simulink model "manual_model_features"  (R2020b)
settings: Solver=VariableStepAuto  StartTime=0.0  StopTime=10.0  RelTol=1e-3
undefined symbols (not defined in the file): sigbuilder_block
libraries: simulink x141
(part 2 of 3)

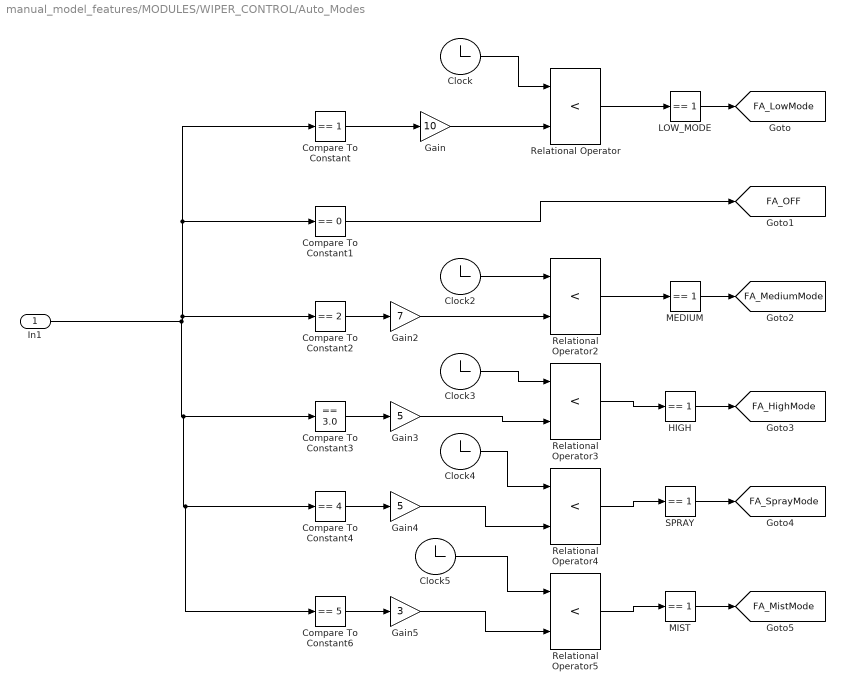
== system manual_model_features/MODULES/WIPER_CONTROL/Auto_Modes ==
  In1 : Inport
  Clock{,2..5} (5 alike) : Clock
      settings: Decimation=5
  Compare To Constant : simulink/Logic and Bit Operations/Compare To Constant  relop===  const=1  OutDataTypeStr=boolean
  Compare To Constant1 : simulink/Logic and Bit Operations/Compare To Constant  relop===  const=0  OutDataTypeStr=boolean
  Compare To Constant2 : simulink/Logic and Bit Operations/Compare To Constant  relop===  const=2  OutDataTypeStr=boolean
  Compare To Constant3 : simulink/Logic and Bit Operations/Compare To Constant  relop===  const=3.0  OutDataTypeStr=boolean
  Compare To Constant4 : simulink/Logic and Bit Operations/Compare To Constant  relop===  const=4  OutDataTypeStr=boolean
  Compare To Constant6 : simulink/Logic and Bit Operations/Compare To Constant  relop===  const=5  OutDataTypeStr=boolean
  Gain : Gain  Gain=10
  Gain2 : Gain  Gain=7
  Gain3 : Gain  Gain=5
  Gain4 : Gain  Gain=5
  Gain5 : Gain  Gain=3
  HIGH : simulink/Logic and Bit Operations/Compare To Constant  relop===  const=1  OutDataTypeStr=boolean
  LOW_MODE : simulink/Logic and Bit Operations/Compare To Constant  relop===  const=1  OutDataTypeStr=boolean
  MEDIUM : simulink/Logic and Bit Operations/Compare To Constant  relop===  const=1  OutDataTypeStr=boolean
  MIST : simulink/Logic and Bit Operations/Compare To Constant  relop===  const=1  OutDataTypeStr=boolean
  Relational Operator{,2..5} (5 alike) : RelationalOperator  Operator=<  OutDataTypeStr=boolean  RndMeth=Simplest
  SPRAY : simulink/Logic and Bit Operations/Compare To Constant  relop===  const=1  OutDataTypeStr=boolean
  tag scope: FA_HighMode=global, FA_LowMode=global, FA_MediumMode=global, FA_MistMode=global, FA_OFF=global, FA_SprayMode=global
  wires:
  In1/1 -> Compare To Constant6/1, Compare To Constant4/1, Compare To Constant3/1, Compare To Constant2/1, Compare To Constant/1, Compare To Constant1/1
  Clock/1 -> Relational Operator/1
  Relational Operator/1 -> LOW_MODE/1
  Gain/1 -> Relational Operator/2
  Compare To Constant/1 -> Gain/1
  Clock2/1 -> Relational Operator2/1
  Gain2/1 -> Relational Operator2/2
  Compare To Constant2/1 -> Gain2/1
  Clock3/1 -> Relational Operator3/1
  Gain3/1 -> Relational Operator3/2
  Compare To Constant3/1 -> Gain3/1
  Gain4/1 -> Relational Operator4/2
  Clock4/1 -> Relational Operator4/1
  Compare To Constant4/1 -> Gain4/1
  LOW_MODE/1 -> [FA_LowMode]
  MEDIUM/1 -> [FA_MediumMode]
  Relational Operator2/1 -> MEDIUM/1
  HIGH/1 -> [FA_HighMode]
  Relational Operator3/1 -> HIGH/1
  SPRAY/1 -> [FA_SprayMode]
  Relational Operator4/1 -> SPRAY/1
  Compare To Constant1/1 -> [FA_OFF]
  Relational Operator5/1 -> MIST/1
  Gain5/1 -> Relational Operator5/2
  Clock5/1 -> Relational Operator5/1
  MIST/1 -> [FA_MistMode]
  Compare To Constant6/1 -> Gain5/1

== system manual_model_features/MODULES/WIPER_CONTROL/Back_Windshield ==
  Lamp : LampBlock

== system manual_model_features/MODULES/WIPER_CONTROL/Front_Windshield ==
  Enable : EnablePort
  Auto_Modes : Subsystem
  Manual_mode : Subsystem
  Rotary Switch : RotarySwitchBlock  Commented=on
      settings: Values={{'Off', 'Low', 'Medium', 'High', 'Spray', 'Manual', 'MistMode'}, [0 1 2 3 4 5 6]}
  wires:
  [FW_Modes] -> Manual_mode/1(In1), Auto_Modes/1(In1)

== system manual_model_features/MODULES/WIPER_CONTROL/Manual_mode ==
  In1 : Inport
  Bw30_60 : Logic  IconShape=distinctive  AllPortsSameDT=off  OutDataTypeStr=boolean
  Bw60_100 : Logic  IconShape=distinctive  AllPortsSameDT=off  OutDataTypeStr=boolean
  Compare To Constant1 : simulink/Logic and Bit Operations/Compare To Constant  relop=>  const=30  OutDataTypeStr=boolean
  Compare To Constant2 : simulink/Logic and Bit Operations/Compare To Constant  relop=<=  const=60  OutDataTypeStr=boolean
  Compare To Constant3 : simulink/Logic and Bit Operations/Compare To Constant  relop=>  const=60  OutDataTypeStr=boolean
  Compare To Constant4 : simulink/Logic and Bit Operations/Compare To Constant  relop=<=  const=100  OutDataTypeStr=boolean
  Display : Display
  LessThan30 : simulink/Logic and Bit Operations/Compare To Constant  relop=<=  const=30  OutDataTypeStr=boolean
  Slider : SliderBlock
  String Constant : StringConstant  String="\"Undefined!\""
  Switch : Switch  Criteria=u2 > Threshold  Threshold=5
  tag scope: FM_Bw30_60=global, FM_Bw60_100=global, FM_lessthan30=global
  wires:
  Compare To Constant1/1 -> Bw30_60/1
  Bw30_60/1 -> [FM_Bw30_60]
  [FC_ManualInput] -> Compare To Constant4/1, Compare To Constant3/1, Compare To Constant2/1, Compare To Constant1/1, LessThan30/1, Switch/1
  Compare To Constant4/1 -> Bw60_100/2
  LessThan30/1 -> [FM_lessthan30]
  Switch/1 -> Display/1
  Compare To Constant3/1 -> Bw60_100/1
  Bw60_100/1 -> [FM_Bw60_100]
  Compare To Constant2/1 -> Bw30_60/2
  In1/1 -> Switch/2
  String Constant/1 -> Switch/3

== system manual_model_features/MODULES/WIPER_CONTROL/Wiper_Control ==
  Inport : Inport
  AND : Logic  IconShape=distinctive  AllPortsSameDT=off  OutDataTypeStr=boolean
  AND1 : Logic  IconShape=distinctive  AllPortsSameDT=off  OutDataTypeStr=boolean
  Atomic Subsystem : Subsystem  TreatAsAtomicUnit=on
  Atomic Subsystem1 : Subsystem  TreatAsAtomicUnit=on
  Back switch : SliderSwitchBlock  Commented=on
      settings: Values={{'Off', 'On'}, [0 1]}
  Back_Windshield : Subsystem  Commented=on  TreatAsAtomicUnit=on
  Front switch : SliderSwitchBlock  Commented=on
      settings: Values={{'Off', 'On'}, [0 1]}
  Front_Windshield : Subsystem  Commented=on  TreatAsAtomicUnit=on
  wires:
  Inport/1 -> AND1/2, AND/2
  [WC_FrontS] -> AND/1
  [WC_BackS] -> AND1/1
  AND1/1 -> Atomic Subsystem/1(Inport)
  AND/1 -> Atomic Subsystem1/1(Inport)

== system manual_model_features/MODULES/system/Automatic_Door_lock ==
  note: roof light
  AND : Logic  IconShape=distinctive  AllPortsSameDT=off  OutDataTypeStr=boolean
  Constant : Constant
  Display : Display
  Display1 : Display
  Display2 : Display
  If : If  IfExpression=u1>=13  ElseIfExpressions=u1<13  ShowElse=off
  If Action Subsystem : Subsystem  TreatAsAtomicUnit=on
  If Action Subsystem1 : Subsystem  TreatAsAtomicUnit=on
  OR : Logic  Operator=OR  IconShape=distinctive  AllPortsSameDT=off  OutDataTypeStr=boolean
  reset : Constant  Value=0
  Out1 : Outport
  wires:
  If Action Subsystem1/1(Out1) -> OR/2
  If Action Subsystem/1(Out1) -> OR/1
  [accln] -> Display/1, If/1
  Constant/1 -> If Action Subsystem/1(In1)
  [ADl_Ignition_System] -> Display1/1, AND/1
  reset/1 -> If Action Subsystem1/1(In1)
  If/2 -> If Action Subsystem1/Action
  If/1 -> If Action Subsystem/Action
  OR/1 -> AND/2
  AND/1 -> Display2/1, Out1/1

== system manual_model_features/MODULES/system/delay system door lock and interior light subsystem ==
  AND : Logic  Inputs=5  IconShape=distinctive  AllPortsSameDT=off  OutDataTypeStr=boolean
  AND1 : Logic  Inputs=4  IconShape=distinctive  AllPortsSameDT=off  OutDataTypeStr=boolean
  Add : Sum
  Compare To Constant : simulink/Logic and Bit Operations/Compare To Constant  relop===  const=0  OutDataTypeStr=boolean
  Constant4 : Constant  Value=0
  Constant5 : Constant  Value=0
  Data Type Conversion : DataTypeConversion
  Delay1 : Delay  DelayLength=1
  Display : Display
  Display1 : Display
  Repeating Sequence Stair : simulink/Sources/Repeating Sequence Stair  OutValues=[1 1]  tsamp=-1  OutMin=[]  OutMax=[]  OutDataTypeStr=double  OutputDataTypeScalingMode=double  OutDataType=fixdt(0,8)  ConRadixGroup=Best Precision: Vector-wise  OutScaling=2^-12
  Scope : Scope
  Switch : Switch  Threshold=5
  Switch1 : Switch
  Out1 : Outport
  tag scope: D_Sys_roof=global
  wires:
  Switch1/1 -> Scope/1, Out1/1, Delay1/1, Display/1
  [D_sys_antilock] -> AND/5
  Repeating Sequence Stair/1 -> Switch1/2
  Delay1/1 -> Add/2
  Constant5/1 -> Switch1/3
  Constant4/1 -> Switch/1
  Add/1 -> Switch/2, Switch/3
  Switch/1 -> Switch1/1
  AND/1 -> Data Type Conversion/1
  [D_sys_Door3] -> AND1/3, AND/3
  [D_sys_Door4] -> AND1/4, AND/4
  AND1/1 -> Compare To Constant/1
  [D_sys_Door1] -> AND1/1, AND/1
  [D_sys_Door2] -> AND1/2, AND/2
  Compare To Constant/1 -> [D_Sys_roof], Display1/1
  Data Type Conversion/1 -> Add/1

== system manual_model_features/MODULES/	POWER_WINDOW/Subsystem4/Front_left_subsystem ==
  lock/unlock : Inport
  In_fl_b : Inport  Port=2
  In_fl_Dc : Inport  Port=3
  object : Inport  Port=4
  Enable : EnablePort
  AND : Logic  IconShape=distinctive  AllPortsSameDT=off  OutDataTypeStr=boolean
  Compare To Constant1 : simulink/Logic and Bit Operations/Compare To Constant  relop===  const=1  OutDataTypeStr=boolean
  Display : Display
  Display1 : Display
  Scope : Scope  NumInputPorts=2
  Switch_lock_unlock : Switch  Criteria=u2 > Threshold
  check_ip : Constant
  decision_Box : Stateflow chart  TreatAsAtomicUnit=on
  inp_data : Logic  Operator=NXOR  IconShape=distinctive  AllPortsSameDT=off  OutDataTypeStr=boolean
  or1 : Logic  Operator=NXOR  IconShape=distinctive  AllPortsSameDT=off  OutDataTypeStr=boolean
  Outport : Outport
  Outport1 : Outport  Port=2
  tag scope: A=global
  wires:
  In_fl_b/1 -> AND/1
  check_ip/1 -> or1/1
  Switch_lock_unlock/1 -> [b1]
  Compare To Constant1/1 -> or1/2
  [b1] -> Display/1
  decision_Box/1(op1) -> Outport1/1, Switch_lock_unlock/3, Switch_lock_unlock/1, Scope/2, [A]
  decision_Box/2(warning) -> Outport/1, Scope/1
  object/1 -> decision_Box/2(data1)
  AND/1 -> inp_data/2  "res"
  or1/1 -> inp_data/1
  lock/unlock/1 -> AND/2, Switch_lock_unlock/2
  [A] -> Display1/1
  inp_data/1 -> decision_Box/1(data)
  In_fl_Dc/1 -> Compare To Constant1/1

== system manual_model_features/MODULES/	POWER_WINDOW/Subsystem4/Rear_right_Subsystem ==
  lock/unlock : Inport
  In2 : Inport  Port=2
  In3 : Inport  Port=3
  object : Inport  Port=4
  Enable : EnablePort
  Chart : Stateflow chart  TreatAsAtomicUnit=on
  Compare To Constant1 : simulink/Logic and Bit Operations/Compare To Constant  relop===  const=3  OutDataTypeStr=boolean
  Constant1 : Constant  Value=3
  Display2 : Display
  Display3 : Display
  Scope : Scope  NumInputPorts=2
  Switch : Switch  Criteria=u2 > Threshold
  or1 : Logic  Operator=NXOR  IconShape=distinctive  AllPortsSameDT=off  OutDataTypeStr=boolean
  or2 : Logic  IconShape=distinctive  AllPortsSameDT=off  OutDataTypeStr=boolean
  or3 : Logic  Operator=NXOR  IconShape=distinctive  AllPortsSameDT=off  OutDataTypeStr=boolean
  Outport : Outport
  Outport1 : Outport  Port=2
  tag scope: c=global
  wires:
  Constant1/1 -> or1/1
  [b3] -> Display2/1
  Compare To Constant1/1 -> or1/2
  Switch/1 -> [b3]
  lock/unlock/1 -> or2/2, Switch/2
  Chart/2(warning) -> Scope/1, Outport/1  "ss3"
  object/1 -> Chart/2(data1)
  or1/1 -> or3/2
  or2/1 -> or3/1  "res"
  or3/1 -> Chart/1(data)
  [c] -> Display3/1
  Chart/1(op1) -> Outport1/1, [c], Scope/2, Switch/3, Switch/1
  In2/1 -> or2/1
  In3/1 -> Compare To Constant1/1

== system manual_model_features/MODULES/	POWER_WINDOW/Subsystem4/driver_control_Subsystem ==
  In1 : Inport
  object : Inport  Port=2
  Enable : EnablePort
  Chart : Stateflow chart  TreatAsAtomicUnit=on
  Display4 : Display
  Scope : Scope  NumInputPorts=2
  Outport : Outport
  Outport1 : Outport  Port=2
  tag scope: d=global
  wires:
  Chart/2(warning) -> Outport/1, Scope/1  "ss4"
  object/1 -> Chart/2(data1)
  In1/1 -> Chart/1(data)
  [d] -> Display4/1
  Chart/1(op1) -> Outport1/1, [d], Scope/2

== system manual_model_features/MODULES/	POWER_WINDOW/Subsystem4/rear_left_Subsystem ==
  lock/unlock : Inport
  In2 : Inport  Port=2
  In3 : Inport  Port=3
  object : Inport  Port=4
  Enable : EnablePort
  Chart : Stateflow chart  TreatAsAtomicUnit=on
  Compare To Constant2 : simulink/Logic and Bit Operations/Compare To Constant  relop===  const=2  OutDataTypeStr=boolean
  Constant1 : Constant  Value=2
  Display1 : Display
  Display2 : Display
  Scope : Scope  NumInputPorts=2
  Switch1 : Switch  Criteria=u2 > Threshold
  or1 : Logic  Operator=NXOR  IconShape=distinctive  AllPortsSameDT=off  OutDataTypeStr=boolean
  or2 : Logic  Operator=NXOR  IconShape=distinctive  AllPortsSameDT=off  OutDataTypeStr=boolean
  or3 : Logic  IconShape=distinctive  AllPortsSameDT=off  OutDataTypeStr=boolean
  Outport : Outport
  Outport1 : Outport  Port=2
  tag scope: b=global
  wires:
  [b2] -> Display1/1
  Constant1/1 -> or2/1
  Compare To Constant2/1 -> or2/2
  Switch1/1 -> [b2]
  lock/unlock/1 -> Switch1/2, or3/2
  object/1 -> Chart/2(data1)
  Chart/2(warning) -> Outport/1, Scope/1  "ss2"
  or3/1 -> or1/1  "res"
  or2/1 -> or1/2
  or1/1 -> Chart/1(data)
  [b] -> Display2/1
  Chart/1(op1) -> Outport1/1, [b], Switch1/3, Switch1/1, Scope/2
  In2/1 -> or3/1
  In3/1 -> Compare To Constant2/1

== system manual_model_features/MODULES/AirBagSystem/FrontAirBagActivation/DriverFrontAirBagActive ==
  In1 : Inport
  Trigger : TriggerPort  VariantControl=(inherit)
  Constant : Constant
  Constant1 : Constant
  Constant2 : Constant
  Relational Operator : RelationalOperator  Operator===  OutDataTypeStr=boolean  RndMeth=Simplest
  Relational Operator1 : RelationalOperator  Operator===  OutDataTypeStr=boolean  RndMeth=Simplest
  Relational Operator2 : RelationalOperator  Operator===  OutDataTypeStr=boolean  RndMeth=Simplest
  tag scope: DriverAB=global, DriverDoor=global, FuelLock=global
  wires:
  In1/1 -> Relational Operator2/1, Relational Operator1/1, Relational Operator/1
  Constant/1 -> Relational Operator/2
  Constant1/1 -> Relational Operator1/2
  Constant2/1 -> Relational Operator2/2
  Relational Operator/1 -> [DriverAB]
  Relational Operator1/1 -> [DriverDoor]
  Relational Operator2/1 -> [FuelLock]

== system manual_model_features/MODULES/AirBagSystem/FrontAirBagActivation/LeftFrontAirBagActive ==
  In2 : Inport
  Trigger : TriggerPort  VariantControl=(inherit)
  Constant : Constant
  Constant1 : Constant
  Constant2 : Constant
  Relational Operator : RelationalOperator  Operator===  OutDataTypeStr=boolean  RndMeth=Simplest
  Relational Operator1 : RelationalOperator  Operator===  OutDataTypeStr=boolean  RndMeth=Simplest
  Relational Operator2 : RelationalOperator  Operator===  OutDataTypeStr=boolean  RndMeth=Simplest
  tag scope: FuelLock1=global, LeftFront=global, LeftFrontDoor=global
  wires:
  Constant1/1 -> Relational Operator1/2
  In2/1 -> Relational Operator2/1, Relational Operator1/1, Relational Operator/1
  Constant2/1 -> Relational Operator2/2
  Constant/1 -> Relational Operator/2
  Relational Operator/1 -> [LeftFront]
  Relational Operator1/1 -> [LeftFrontDoor]
  Relational Operator2/1 -> [FuelLock1]

== system manual_model_features/MODULES/AirBagSystem/FrontAirBagActivation/LeftRearAirBagActive ==
  In1 : Inport
  Trigger : TriggerPort  VariantControl=(inherit)
  Constant : Constant
  Constant1 : Constant
  Constant2 : Constant
  Relational Operator : RelationalOperator  Operator===  OutDataTypeStr=boolean  RndMeth=Simplest
  Relational Operator1 : RelationalOperator  Operator===  OutDataTypeStr=boolean  RndMeth=Simplest
  Relational Operator2 : RelationalOperator  Operator===  OutDataTypeStr=boolean  RndMeth=Simplest
  tag scope: FuelLock2=global, RearLeft=global, RearLeftDoor=global
  wires:
  Constant1/1 -> Relational Operator1/2
  In1/1 -> Relational Operator2/1, Relational Operator1/1, Relational Operator/1
  Constant2/1 -> Relational Operator2/2
  Constant/1 -> Relational Operator/2
  Relational Operator/1 -> [RearLeft]
  Relational Operator1/1 -> [RearLeftDoor]
  Relational Operator2/1 -> [FuelLock2]

== system manual_model_features/MODULES/AirBagSystem/FrontAirBagActivation/RightRearAirBagActive ==
  In2 : Inport
  Trigger : TriggerPort  VariantControl=(inherit)
  Constant : Constant
  Constant1 : Constant
  Constant2 : Constant
  Relational Operator : RelationalOperator  Operator===  OutDataTypeStr=boolean  RndMeth=Simplest
  Relational Operator1 : RelationalOperator  Operator===  OutDataTypeStr=boolean  RndMeth=Simplest
  Relational Operator2 : RelationalOperator  Operator===  OutDataTypeStr=boolean  RndMeth=Simplest
  tag scope: FuelLock3=global, RearRight=global, RearRightDoor=global
  wires:
  Constant1/1 -> Relational Operator1/2
  In2/1 -> Relational Operator2/1, Relational Operator1/1, Relational Operator/1
  Constant2/1 -> Relational Operator2/2
  Constant/1 -> Relational Operator/2
  Relational Operator/1 -> [RearRight]
  Relational Operator1/1 -> [RearRightDoor]
  Relational Operator2/1 -> [FuelLock3]

== system manual_model_features/MODULES/AirBagSystem/SideAirBagActivation/DriverSideAirBagActive ==
  In1 : Inport
  Trigger : TriggerPort  VariantControl=(inherit)
  Constant : Constant
  Constant1 : Constant
  Constant2 : Constant
  Relational Operator : RelationalOperator  Operator===  OutDataTypeStr=boolean  RndMeth=Simplest
  Relational Operator1 : RelationalOperator  Operator===  OutDataTypeStr=boolean  RndMeth=Simplest
  Relational Operator2 : RelationalOperator  Operator===  OutDataTypeStr=boolean  RndMeth=Simplest
  tag scope: DriverABSide=global, DriverDoorSide=global, FuelLockSide=global
  wires:
  In1/1 -> Relational Operator2/1, Relational Operator1/1, Relational Operator/1
  Constant/1 -> Relational Operator/2
  Constant1/1 -> Relational Operator1/2
  Constant2/1 -> Relational Operator2/2
  Relational Operator/1 -> [DriverABSide]
  Relational Operator1/1 -> [DriverDoorSide]
  Relational Operator2/1 -> [FuelLockSide]

== system manual_model_features/MODULES/AirBagSystem/SideAirBagActivation/LeftFronrSeatAirBagActive ==
  In2 : Inport
  Trigger : TriggerPort  VariantControl=(inherit)
  Constant : Constant
  Constant1 : Constant
  Constant2 : Constant
  Relational Operator : RelationalOperator  Operator===  OutDataTypeStr=boolean  RndMeth=Simplest
  Relational Operator1 : RelationalOperator  Operator===  OutDataTypeStr=boolean  RndMeth=Simplest
  Relational Operator2 : RelationalOperator  Operator===  OutDataTypeStr=boolean  RndMeth=Simplest
  tag scope: FuelLockSide1=global, LeftFrontDoorSide=global, LeftFrontSide=global
  wires:
  Constant1/1 -> Relational Operator1/2
  In2/1 -> Relational Operator2/1, Relational Operator1/1, Relational Operator/1
  Constant2/1 -> Relational Operator2/2
  Constant/1 -> Relational Operator/2
  Relational Operator/1 -> [LeftFrontSide]
  Relational Operator1/1 -> [LeftFrontDoorSide]
  Relational Operator2/1 -> [FuelLockSide1]

== system manual_model_features/MODULES/AirBagSystem/SideAirBagActivation/LeftRearAirBagActive ==
  In1 : Inport
  Trigger : TriggerPort  VariantControl=(inherit)
  Constant : Constant
  Constant1 : Constant
  Constant2 : Constant
  Relational Operator : RelationalOperator  Operator===  OutDataTypeStr=boolean  RndMeth=Simplest
  Relational Operator1 : RelationalOperator  Operator===  OutDataTypeStr=boolean  RndMeth=Simplest
  Relational Operator2 : RelationalOperator  Operator===  OutDataTypeStr=boolean  RndMeth=Simplest
  tag scope: FuelLockSide2=global, RearLeftDoorSide=global, RearLeftSide=global
  wires:
  Constant1/1 -> Relational Operator1/2
  In1/1 -> Relational Operator2/1, Relational Operator1/1, Relational Operator/1
  Constant2/1 -> Relational Operator2/2
  Constant/1 -> Relational Operator/2
  Relational Operator1/1 -> [RearLeftDoorSide]
  Relational Operator2/1 -> [FuelLockSide2]
  Relational Operator/1 -> [RearLeftSide]

== system manual_model_features/MODULES/AirBagSystem/SideAirBagActivation/RightRearAirBagActive ==
  In2 : Inport
  Trigger : TriggerPort  VariantControl=(inherit)
  Constant : Constant
  Constant1 : Constant
  Constant2 : Constant
  Relational Operator : RelationalOperator  Operator===  OutDataTypeStr=boolean  RndMeth=Simplest
  Relational Operator1 : RelationalOperator  Operator===  OutDataTypeStr=boolean  RndMeth=Simplest
  Relational Operator2 : RelationalOperator  Operator===  OutDataTypeStr=boolean  RndMeth=Simplest
  tag scope: FuelLockSide3=global, RearRightDoorSide=global, RearRightSide=global
  wires:
  Constant1/1 -> Relational Operator1/2
  In2/1 -> Relational Operator2/1, Relational Operator1/1, Relational Operator/1
  Constant2/1 -> Relational Operator2/2
  Constant/1 -> Relational Operator/2
  Relational Operator/1 -> [RearRightSide]
  Relational Operator1/1 -> [RearRightDoorSide]
  Relational Operator2/1 -> [FuelLockSide3]

== system manual_model_features/MODULES/AirBagSystem2/FrontAirBagActivation/DriverFrontAirBagActive ==
  In1 : Inport
  Trigger : TriggerPort  VariantControl=(inherit)
  Constant : Constant
  Constant1 : Constant
  Constant2 : Constant
  DriverDoorUnlock : LampBlock
  DriverFront : LampBlock
  FuelLock : LampBlock
  Relational Operator : RelationalOperator  Operator===  OutDataTypeStr=boolean  RndMeth=Simplest
  Relational Operator1 : RelationalOperator  Operator===  OutDataTypeStr=boolean  RndMeth=Simplest
  Relational Operator2 : RelationalOperator  Operator===  OutDataTypeStr=boolean  RndMeth=Simplest
  wires:
  In1/1 -> Relational Operator2/1, Relational Operator1/1, Relational Operator/1
  Constant/1 -> Relational Operator/2
  Constant1/1 -> Relational Operator1/2
  Constant2/1 -> Relational Operator2/2

== system manual_model_features/MODULES/AirBagSystem2/FrontAirBagActivation/LeftFrontAirBagActive ==
  In2 : Inport
  Trigger : TriggerPort  VariantControl=(inherit)
  Constant : Constant
  Constant1 : Constant
  Constant2 : Constant
  FuelLock : LampBlock
  LeftDoorUnlock : LampBlock
  LeftFront : LampBlock
  Relational Operator : RelationalOperator  Operator===  OutDataTypeStr=boolean  RndMeth=Simplest
  Relational Operator1 : RelationalOperator  Operator===  OutDataTypeStr=boolean  RndMeth=Simplest
  Relational Operator2 : RelationalOperator  Operator===  OutDataTypeStr=boolean  RndMeth=Simplest
  wires:
  Constant1/1 -> Relational Operator1/2
  In2/1 -> Relational Operator2/1, Relational Operator1/1, Relational Operator/1
  Constant2/1 -> Relational Operator2/2
  Constant/1 -> Relational Operator/2

== system manual_model_features/MODULES/AirBagSystem2/FrontAirBagActivation/LeftRearAirBagActive ==
  In1 : Inport
  Trigger : TriggerPort  VariantControl=(inherit)
  Constant : Constant
  Constant1 : Constant
  Constant2 : Constant
  FuelLock : LampBlock
  LeftRear : LampBlock
  LeftRearDoorUnlock : LampBlock
  Relational Operator : RelationalOperator  Operator===  OutDataTypeStr=boolean  RndMeth=Simplest
  Relational Operator1 : RelationalOperator  Operator===  OutDataTypeStr=boolean  RndMeth=Simplest
  Relational Operator2 : RelationalOperator  Operator===  OutDataTypeStr=boolean  RndMeth=Simplest
  wires:
  Constant1/1 -> Relational Operator1/2
  In1/1 -> Relational Operator2/1, Relational Operator1/1, Relational Operator/1
  Constant2/1 -> Relational Operator2/2
  Constant/1 -> Relational Operator/2

== system manual_model_features/MODULES/AirBagSystem2/FrontAirBagActivation/RightRearAirBagActive ==
  In2 : Inport
  Trigger : TriggerPort  VariantControl=(inherit)
  Constant : Constant
  Constant1 : Constant
  Constant2 : Constant
  FuelLock : LampBlock
  Relational Operator : RelationalOperator  Operator===  OutDataTypeStr=boolean  RndMeth=Simplest
  Relational Operator1 : RelationalOperator  Operator===  OutDataTypeStr=boolean  RndMeth=Simplest
  Relational Operator2 : RelationalOperator  Operator===  OutDataTypeStr=boolean  RndMeth=Simplest
  RightRear : LampBlock
  RightRearDoorUnlock : LampBlock
  wires:
  Constant1/1 -> Relational Operator1/2
  In2/1 -> Relational Operator2/1, Relational Operator1/1, Relational Operator/1
  Constant2/1 -> Relational Operator2/2
  Constant/1 -> Relational Operator/2

== system manual_model_features/MODULES/AirBagSystem2/FrontAirBagActivation1/DriverSideAirBagActive ==
  In1 : Inport
  Trigger : TriggerPort  VariantControl=(inherit)
  Constant : Constant
  Constant1 : Constant
  Constant2 : Constant
  DriverDoorUnlock : LampBlock
  DriverFront : LampBlock
  FuelLock : LampBlock
  Relational Operator : RelationalOperator  Operator===  OutDataTypeStr=boolean  RndMeth=Simplest
  Relational Operator1 : RelationalOperator  Operator===  OutDataTypeStr=boolean  RndMeth=Simplest
  Relational Operator2 : RelationalOperator  Operator===  OutDataTypeStr=boolean  RndMeth=Simplest
  Out1 : Outport
  wires:
  In1/1 -> Relational Operator2/1, Relational Operator1/1, Relational Operator/1
  Constant/1 -> Relational Operator/2
  Constant1/1 -> Relational Operator1/2
  Constant2/1 -> Relational Operator2/2

== system manual_model_features/MODULES/AirBagSystem2/FrontAirBagActivation1/LeftFronrSeatAirBagActive ==
  In2 : Inport
  Trigger : TriggerPort  VariantControl=(inherit)
  Constant : Constant
  Constant1 : Constant
  Constant2 : Constant
  FuelLock : LampBlock
  LeftDoorUnlock : LampBlock
  LeftFront : LampBlock
  Relational Operator : RelationalOperator  Operator===  OutDataTypeStr=boolean  RndMeth=Simplest
  Relational Operator1 : RelationalOperator  Operator===  OutDataTypeStr=boolean  RndMeth=Simplest
  Relational Operator2 : RelationalOperator  Operator===  OutDataTypeStr=boolean  RndMeth=Simplest
  wires:
  Constant1/1 -> Relational Operator1/2
  In2/1 -> Relational Operator2/1, Relational Operator1/1, Relational Operator/1
  Constant2/1 -> Relational Operator2/2
  Constant/1 -> Relational Operator/2

== system manual_model_features/MODULES/AirBagSystem2/FrontAirBagActivation1/LeftRearAirBagActive ==
  In1 : Inport
  Trigger : TriggerPort  VariantControl=(inherit)
  Constant : Constant
  Constant1 : Constant
  Constant2 : Constant
  FuelLock : LampBlock
  LeftRear : LampBlock
  LeftRearDoorUnlock : LampBlock
  Relational Operator : RelationalOperator  Operator===  OutDataTypeStr=boolean  RndMeth=Simplest
  Relational Operator1 : RelationalOperator  Operator===  OutDataTypeStr=boolean  RndMeth=Simplest
  Relational Operator2 : RelationalOperator  Operator===  OutDataTypeStr=boolean  RndMeth=Simplest
  wires:
  Constant1/1 -> Relational Operator1/2
  In1/1 -> Relational Operator2/1, Relational Operator1/1, Relational Operator/1
  Constant2/1 -> Relational Operator2/2
  Constant/1 -> Relational Operator/2

== system manual_model_features/MODULES/AirBagSystem2/FrontAirBagActivation1/RightRearAirBagActive ==
  In2 : Inport
  Trigger : TriggerPort  VariantControl=(inherit)
  Constant : Constant
  Constant1 : Constant
  Constant2 : Constant
  FuelLock : LampBlock
  Relational Operator : RelationalOperator  Operator===  OutDataTypeStr=boolean  RndMeth=Simplest
  Relational Operator1 : RelationalOperator  Operator===  OutDataTypeStr=boolean  RndMeth=Simplest
  Relational Operator2 : RelationalOperator  Operator===  OutDataTypeStr=boolean  RndMeth=Simplest
  RightRear : LampBlock
  RightRearDoorUnlock : LampBlock
  wires:
  Constant1/1 -> Relational Operator1/2
  In2/1 -> Relational Operator2/1, Relational Operator1/1, Relational Operator/1
  Constant2/1 -> Relational Operator2/2
  Constant/1 -> Relational Operator/2

== system manual_model_features/MODULES/Door_System/AutomaticDoorLock/If Action Subsystem ==
  In1 : Inport
  Action Port : ActionPort
  Out1 : Outport
  wires:
  In1/1 -> Out1/1

== system manual_model_features/MODULES/Door_System/AutomaticDoorLock/If Action Subsystem1 ==
  In1 : Inport
  Action Port : ActionPort
  Out1 : Outport
  wires:
  In1/1 -> Out1/1

== system manual_model_features/MODULES/SeatRestraintSystem1/PowerLumbar/PowerSeat ==
  RearAdjust : Inport
  SeatAdjust : Inport  Port=2
  CushionAdjust : Inport  Port=3
  Enable : EnablePort
  ModeSelection==RearAdjust : Constant  Value=2
  Subsystem : Subsystem
  Subsystem1 : Subsystem
  Subsystem2 : Subsystem
  wires:
  RearAdjust/1 -> Subsystem/1(Rear_Adjust)
  ModeSelection==RearAdjust/1 -> Subsystem2/1(Mode_Check), Subsystem1/1(Mode_Check), Subsystem/2(Mode_Check)
  SeatAdjust/1 -> Subsystem1/2(Seat_Adjust)
  CushionAdjust/1 -> Subsystem2/2(CushionAdjust)

== system manual_model_features/MODULES/Subsystem2/Subsystem/Enabled Subsystem ==
  In1 : Inport
  Enable : EnablePort
  Outport : Outport
  wires:
  In1/1 -> Outport/1

== system manual_model_features/MODULES/Subsystem2/Subsystem1/Enabled Subsystem1 ==
  In1 : Inport
  Enable : EnablePort
  Outport : Outport
  wires:
  In1/1 -> Outport/1

== system manual_model_features/MODULES/Tire Pressure Monitoring System/TP_Monitoring/indicateHigh1 ==
  Enable : EnablePort
  Constant : Constant  Value=0
  Out1 : Outport
  wires:
  Constant/1 -> Out1/1

== system manual_model_features/MODULES/Tire Pressure Monitoring System/TP_Monitoring/indicateHigh2 ==
  Enable : EnablePort
  Constant : Constant  Value=0
  Out1 : Outport
  wires:
  Constant/1 -> Out1/1

== system manual_model_features/MODULES/Tire Pressure Monitoring System/TP_Monitoring/indicateHigh3 ==
  Enable : EnablePort
  Constant : Constant  Value=0
  Out1 : Outport
  wires:
  Constant/1 -> Out1/1

== system manual_model_features/MODULES/Tire Pressure Monitoring System/TP_Monitoring/indicateHigh4 ==
  Enable : EnablePort
  Constant : Constant  Value=0
  Out1 : Outport
  wires:
  Constant/1 -> Out1/1

== system manual_model_features/MODULES/Tire Pressure Monitoring System/TP_Monitoring/indicateLow1 ==
  Enable : EnablePort
  Constant : Constant
  Out1 : Outport
  wires:
  Constant/1 -> Out1/1

== system manual_model_features/MODULES/Tire Pressure Monitoring System/TP_Monitoring/indicateLow2 ==
  Enable : EnablePort
  Constant : Constant
  Out1 : Outport
  wires:
  Constant/1 -> Out1/1

== system manual_model_features/MODULES/Tire Pressure Monitoring System/TP_Monitoring/indicateLow3 ==
  Enable : EnablePort
  Constant : Constant
  Out1 : Outport
  wires:
  Constant/1 -> Out1/1

== system manual_model_features/MODULES/Tire Pressure Monitoring System/TP_Monitoring/indicateLow4 ==
  Enable : EnablePort
  Constant : Constant
  Out1 : Outport
  wires:
  Constant/1 -> Out1/1

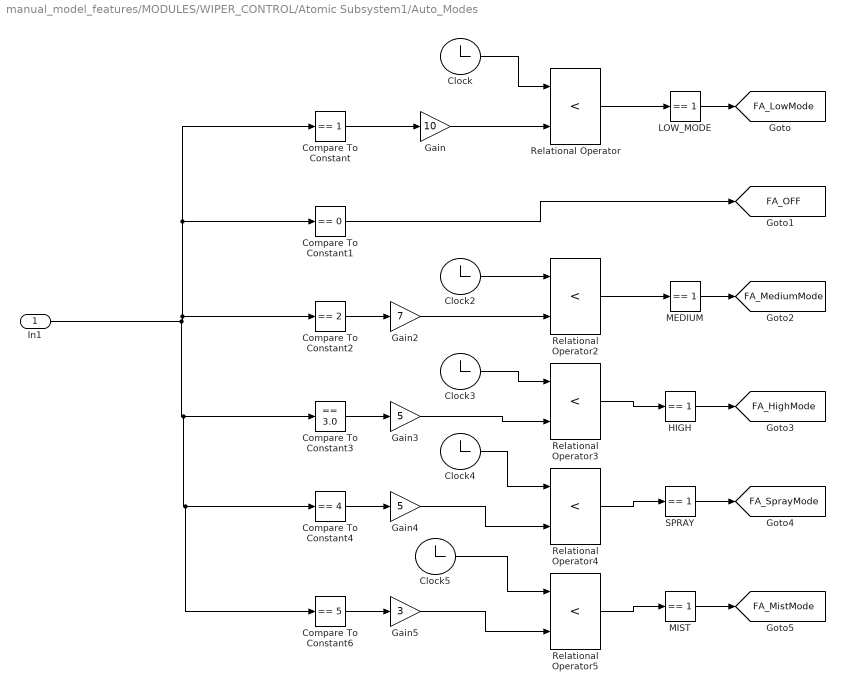
== system manual_model_features/MODULES/WIPER_CONTROL/Atomic Subsystem1/Auto_Modes ==
  In1 : Inport
  Clock{,2..5} (5 alike) : Clock
      settings: Decimation=5
  Compare To Constant : simulink/Logic and Bit Operations/Compare To Constant  relop===  const=1  OutDataTypeStr=boolean
  Compare To Constant1 : simulink/Logic and Bit Operations/Compare To Constant  relop===  const=0  OutDataTypeStr=boolean
  Compare To Constant2 : simulink/Logic and Bit Operations/Compare To Constant  relop===  const=2  OutDataTypeStr=boolean
  Compare To Constant3 : simulink/Logic and Bit Operations/Compare To Constant  relop===  const=3.0  OutDataTypeStr=boolean
  Compare To Constant4 : simulink/Logic and Bit Operations/Compare To Constant  relop===  const=4  OutDataTypeStr=boolean
  Compare To Constant6 : simulink/Logic and Bit Operations/Compare To Constant  relop===  const=5  OutDataTypeStr=boolean
  Gain : Gain  Gain=10
  Gain2 : Gain  Gain=7
  Gain3 : Gain  Gain=5
  Gain4 : Gain  Gain=5
  Gain5 : Gain  Gain=3
  HIGH : simulink/Logic and Bit Operations/Compare To Constant  relop===  const=1  OutDataTypeStr=boolean
  LOW_MODE : simulink/Logic and Bit Operations/Compare To Constant  relop===  const=1  OutDataTypeStr=boolean
  MEDIUM : simulink/Logic and Bit Operations/Compare To Constant  relop===  const=1  OutDataTypeStr=boolean
  MIST : simulink/Logic and Bit Operations/Compare To Constant  relop===  const=1  OutDataTypeStr=boolean
  Relational Operator{,2..5} (5 alike) : RelationalOperator  Operator=<  OutDataTypeStr=boolean  RndMeth=Simplest
  SPRAY : simulink/Logic and Bit Operations/Compare To Constant  relop===  const=1  OutDataTypeStr=boolean
  tag scope: FA_HighMode=global, FA_LowMode=global, FA_MediumMode=global, FA_MistMode=global, FA_OFF=global, FA_SprayMode=global
  wires:
  In1/1 -> Compare To Constant6/1, Compare To Constant4/1, Compare To Constant3/1, Compare To Constant2/1, Compare To Constant/1, Compare To Constant1/1
  Clock/1 -> Relational Operator/1
  Relational Operator/1 -> LOW_MODE/1
  Gain/1 -> Relational Operator/2
  Compare To Constant/1 -> Gain/1
  Clock2/1 -> Relational Operator2/1
  Gain2/1 -> Relational Operator2/2
  Compare To Constant2/1 -> Gain2/1
  Clock3/1 -> Relational Operator3/1
  Gain3/1 -> Relational Operator3/2
  Compare To Constant3/1 -> Gain3/1
  Gain4/1 -> Relational Operator4/2
  Clock4/1 -> Relational Operator4/1
  Compare To Constant4/1 -> Gain4/1
  LOW_MODE/1 -> [FA_LowMode]
  MEDIUM/1 -> [FA_MediumMode]
  Relational Operator2/1 -> MEDIUM/1
  HIGH/1 -> [FA_HighMode]
  Relational Operator3/1 -> HIGH/1
  SPRAY/1 -> [FA_SprayMode]
  Relational Operator4/1 -> SPRAY/1
  Compare To Constant1/1 -> [FA_OFF]
  Relational Operator5/1 -> MIST/1
  Gain5/1 -> Relational Operator5/2
  Clock5/1 -> Relational Operator5/1
  MIST/1 -> [FA_MistMode]
  Compare To Constant6/1 -> Gain5/1

== system manual_model_features/MODULES/WIPER_CONTROL/Atomic Subsystem1/Manual_mode ==
  In1 : Inport
  Bw30_60 : Logic  IconShape=distinctive  AllPortsSameDT=off  OutDataTypeStr=boolean
  Bw60_100 : Logic  IconShape=distinctive  AllPortsSameDT=off  OutDataTypeStr=boolean
  Compare To Constant1 : simulink/Logic and Bit Operations/Compare To Constant  relop=>  const=30  OutDataTypeStr=boolean
  Compare To Constant2 : simulink/Logic and Bit Operations/Compare To Constant  relop=<=  const=60  OutDataTypeStr=boolean
  Compare To Constant3 : simulink/Logic and Bit Operations/Compare To Constant  relop=>  const=60  OutDataTypeStr=boolean
  Compare To Constant4 : simulink/Logic and Bit Operations/Compare To Constant  relop=<=  const=100  OutDataTypeStr=boolean
  Display : Display
  LessThan30 : simulink/Logic and Bit Operations/Compare To Constant  relop=<=  const=30  OutDataTypeStr=boolean
  Slider : SliderBlock
  String Constant : StringConstant  String="\"Undefined!\""
  Switch : Switch  Criteria=u2 > Threshold  Threshold=5
  tag scope: FM_Bw30_60=global, FM_Bw60_100=global, FM_lessthan30=global
  wires:
  Compare To Constant1/1 -> Bw30_60/1
  Bw30_60/1 -> [FM_Bw30_60]
  [FC_ManualInput] -> Compare To Constant4/1, Compare To Constant3/1, Compare To Constant2/1, Compare To Constant1/1, LessThan30/1, Switch/1
  Compare To Constant4/1 -> Bw60_100/2
  LessThan30/1 -> [FM_lessthan30]
  Switch/1 -> Display/1
  Compare To Constant3/1 -> Bw60_100/1
  Bw60_100/1 -> [FM_Bw60_100]
  Compare To Constant2/1 -> Bw30_60/2
  In1/1 -> Switch/2
  String Constant/1 -> Switch/3

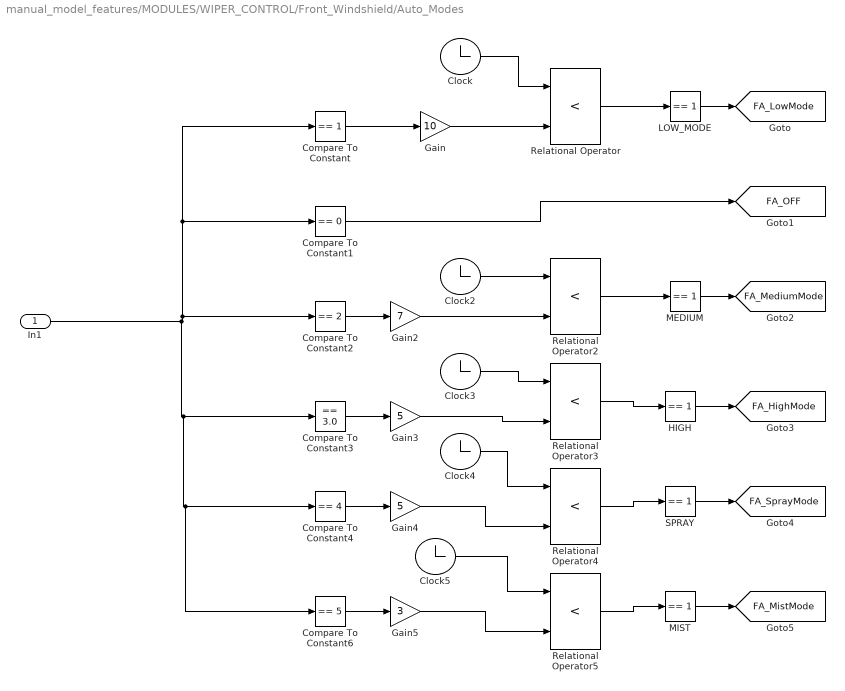
== system manual_model_features/MODULES/WIPER_CONTROL/Front_Windshield/Auto_Modes ==
  In1 : Inport
  Clock{,2..5} (5 alike) : Clock
      settings: Decimation=5
  Compare To Constant : simulink/Logic and Bit Operations/Compare To Constant  relop===  const=1  OutDataTypeStr=boolean
  Compare To Constant1 : simulink/Logic and Bit Operations/Compare To Constant  relop===  const=0  OutDataTypeStr=boolean
  Compare To Constant2 : simulink/Logic and Bit Operations/Compare To Constant  relop===  const=2  OutDataTypeStr=boolean
  Compare To Constant3 : simulink/Logic and Bit Operations/Compare To Constant  relop===  const=3.0  OutDataTypeStr=boolean
  Compare To Constant4 : simulink/Logic and Bit Operations/Compare To Constant  relop===  const=4  OutDataTypeStr=boolean
  Compare To Constant6 : simulink/Logic and Bit Operations/Compare To Constant  relop===  const=5  OutDataTypeStr=boolean
  Gain : Gain  Gain=10
  Gain2 : Gain  Gain=7
  Gain3 : Gain  Gain=5
  Gain4 : Gain  Gain=5
  Gain5 : Gain  Gain=3
  HIGH : simulink/Logic and Bit Operations/Compare To Constant  relop===  const=1  OutDataTypeStr=boolean
  LOW_MODE : simulink/Logic and Bit Operations/Compare To Constant  relop===  const=1  OutDataTypeStr=boolean
  MEDIUM : simulink/Logic and Bit Operations/Compare To Constant  relop===  const=1  OutDataTypeStr=boolean
  MIST : simulink/Logic and Bit Operations/Compare To Constant  relop===  const=1  OutDataTypeStr=boolean
  Relational Operator{,2..5} (5 alike) : RelationalOperator  Operator=<  OutDataTypeStr=boolean  RndMeth=Simplest
  SPRAY : simulink/Logic and Bit Operations/Compare To Constant  relop===  const=1  OutDataTypeStr=boolean
  tag scope: FA_HighMode=global, FA_LowMode=global, FA_MediumMode=global, FA_MistMode=global, FA_OFF=global, FA_SprayMode=global
  wires:
  In1/1 -> Compare To Constant6/1, Compare To Constant4/1, Compare To Constant3/1, Compare To Constant2/1, Compare To Constant/1, Compare To Constant1/1
  Clock/1 -> Relational Operator/1
  Relational Operator/1 -> LOW_MODE/1
  Gain/1 -> Relational Operator/2
  Compare To Constant/1 -> Gain/1
  Clock2/1 -> Relational Operator2/1
  Gain2/1 -> Relational Operator2/2
  Compare To Constant2/1 -> Gain2/1
  Clock3/1 -> Relational Operator3/1
  Gain3/1 -> Relational Operator3/2
  Compare To Constant3/1 -> Gain3/1
  Gain4/1 -> Relational Operator4/2
  Clock4/1 -> Relational Operator4/1
  Compare To Constant4/1 -> Gain4/1
  LOW_MODE/1 -> [FA_LowMode]
  MEDIUM/1 -> [FA_MediumMode]
  Relational Operator2/1 -> MEDIUM/1
  HIGH/1 -> [FA_HighMode]
  Relational Operator3/1 -> HIGH/1
  SPRAY/1 -> [FA_SprayMode]
  Relational Operator4/1 -> SPRAY/1
  Compare To Constant1/1 -> [FA_OFF]
  Relational Operator5/1 -> MIST/1
  Gain5/1 -> Relational Operator5/2
  Clock5/1 -> Relational Operator5/1
  MIST/1 -> [FA_MistMode]
  Compare To Constant6/1 -> Gain5/1

== system manual_model_features/MODULES/WIPER_CONTROL/Front_Windshield/Manual_mode ==
  In1 : Inport
  Bw30_60 : Logic  IconShape=distinctive  AllPortsSameDT=off  OutDataTypeStr=boolean
  Bw60_100 : Logic  IconShape=distinctive  AllPortsSameDT=off  OutDataTypeStr=boolean
  Compare To Constant1 : simulink/Logic and Bit Operations/Compare To Constant  relop=>  const=30  OutDataTypeStr=boolean
  Compare To Constant2 : simulink/Logic and Bit Operations/Compare To Constant  relop=<=  const=60  OutDataTypeStr=boolean
  Compare To Constant3 : simulink/Logic and Bit Operations/Compare To Constant  relop=>  const=60  OutDataTypeStr=boolean
  Compare To Constant4 : simulink/Logic and Bit Operations/Compare To Constant  relop=<=  const=100  OutDataTypeStr=boolean
  Display : Display
  LessThan30 : simulink/Logic and Bit Operations/Compare To Constant  relop=<=  const=30  OutDataTypeStr=boolean
  Slider : SliderBlock
  String Constant : StringConstant  String="\"Undefined!\""
  Switch : Switch  Criteria=u2 > Threshold  Threshold=5
  tag scope: FM_Bw30_60=global, FM_Bw60_100=global, FM_lessthan30=global
  wires:
  Compare To Constant1/1 -> Bw30_60/1
  Bw30_60/1 -> [FM_Bw30_60]
  [FC_ManualInput] -> Compare To Constant4/1, Compare To Constant3/1, Compare To Constant2/1, Compare To Constant1/1, LessThan30/1, Switch/1
  Compare To Constant4/1 -> Bw60_100/2
  LessThan30/1 -> [FM_lessthan30]
  Switch/1 -> Display/1
  Compare To Constant3/1 -> Bw60_100/1
  Bw60_100/1 -> [FM_Bw60_100]
  Compare To Constant2/1 -> Bw30_60/2
  In1/1 -> Switch/2
  String Constant/1 -> Switch/3

== system manual_model_features/MODULES/WIPER_CONTROL/Wiper_Control/Atomic Subsystem ==
  Inport : Inport
  Clock : Clock
      settings: Decimation=5
  Compare To Constant : simulink/Logic and Bit Operations/Compare To Constant  relop===  const=1  OutDataTypeStr=boolean
  Compare To Constant5 : simulink/Logic and Bit Operations/Compare To Constant  relop===  const=1  OutDataTypeStr=boolean
  Gain : Gain  Gain=10
  Relational Operator : RelationalOperator  Operator=<  OutDataTypeStr=boolean  RndMeth=Simplest
  tag scope: BW_Display=global
  wires:
  Compare To Constant5/1 -> [BW_Display]
  Inport/1 -> Compare To Constant/1
  Gain/1 -> Relational Operator/2
  Clock/1 -> Relational Operator/1
  Relational Operator/1 -> Compare To Constant5/1
  Compare To Constant/1 -> Gain/1

== system manual_model_features/MODULES/WIPER_CONTROL/Wiper_Control/Atomic Subsystem1 ==
  Inport : Inport
  Auto_Modes : Subsystem
  Display : Display
  Manual_mode : Subsystem
  wires:
  [FW_Modes] -> Manual_mode/1(In1), Auto_Modes/1(In1)
  Inport/1 -> Display/1

== system manual_model_features/MODULES/WIPER_CONTROL/Wiper_Control/Back_Windshield ==
  Lamp : LampBlock

== system manual_model_features/MODULES/WIPER_CONTROL/Wiper_Control/Front_Windshield ==
  Enable : EnablePort
  Auto_Modes : Subsystem
  Manual_mode : Subsystem
  Rotary Switch : RotarySwitchBlock  Commented=on
      settings: Values={{'Off', 'Low', 'Medium', 'High', 'Spray', 'Manual', 'MistMode'}, [0 1 2 3 4 5 6]}
  wires:
  [FW_Modes] -> Manual_mode/1(In1), Auto_Modes/1(In1)

== system manual_model_features/MODULES/system/Automatic_Door_lock/If Action Subsystem ==
  In1 : Inport
  Action Port : ActionPort
  Out1 : Outport
  wires:
  In1/1 -> Out1/1

== system manual_model_features/MODULES/system/Automatic_Door_lock/If Action Subsystem1 ==
  In1 : Inport
  Action Port : ActionPort
  Out1 : Outport
  wires:
  In1/1 -> Out1/1

== system manual_model_features/MODULES/SeatRestraintSystem1/PowerLumbar/PowerSeat/Subsystem ==
  Rear_Adjust : Inport
  Mode_Check : Inport  Port=2
  AND : Logic  IconShape=distinctive  AllPortsSameDT=off  OutDataTypeStr=boolean
  Constant : Constant
  RearAdjustMode : Constant
  RearAdjustmentLogic : Subsystem  TreatAsAtomicUnit=on
  Relational Operator : RelationalOperator  Operator===  OutDataTypeStr=boolean  RndMeth=Simplest
  Relational Operator1 : RelationalOperator  Operator===  OutDataTypeStr=boolean  RndMeth=Simplest
  wires:
  RearAdjustMode/1 -> Relational Operator/1
  Rear_Adjust/1 -> AND/2
  Constant/1 -> Relational Operator1/2
  Relational Operator1/1 -> RearAdjustmentLogic/Enable, RearAdjustmentLogic/1(ConditionCheck)
  Mode_Check/1 -> Relational Operator/2
  AND/1 -> Relational Operator1/1
  Relational Operator/1 -> AND/1

== system manual_model_features/MODULES/SeatRestraintSystem1/PowerLumbar/PowerSeat/Subsystem1 ==
  Mode_Check : Inport
  Seat_Adjust : Inport  Port=2
  AND1 : Logic  IconShape=distinctive  AllPortsSameDT=off  OutDataTypeStr=boolean
  Constant1 : Constant
  Relational Operator3 : RelationalOperator  Operator===  OutDataTypeStr=boolean  RndMeth=Simplest
  Relational Operator4 : RelationalOperator  Operator===  OutDataTypeStr=boolean  RndMeth=Simplest
  SeatAdjustMode : Constant
  SeatAdjustmentLogic : Subsystem  TreatAsAtomicUnit=on
  wires:
  Constant1/1 -> Relational Operator4/2
  Relational Operator4/1 -> SeatAdjustmentLogic/1(ConditionCheck), SeatAdjustmentLogic/Enable
  Relational Operator3/1 -> AND1/1
  AND1/1 -> Relational Operator4/1
  SeatAdjustMode/1 -> Relational Operator3/2
  Seat_Adjust/1 -> AND1/2
  Mode_Check/1 -> Relational Operator3/1

== system manual_model_features/MODULES/SeatRestraintSystem1/PowerLumbar/PowerSeat/Subsystem2 ==
  Mode_Check : Inport
  CushionAdjust : Inport  Port=2
  AND2 : Logic  IconShape=distinctive  AllPortsSameDT=off  OutDataTypeStr=boolean
  Constant2 : Constant
  CushionAdjustMode : Constant  Value=2
  CushionAdjustmentLogic : Subsystem  TreatAsAtomicUnit=on
  Relational Operator2 : RelationalOperator  Operator===  OutDataTypeStr=boolean  RndMeth=Simplest
  Relational Operator5 : RelationalOperator  Operator===  OutDataTypeStr=boolean  RndMeth=Simplest
  wires:
  Relational Operator5/1 -> CushionAdjustmentLogic/Enable, CushionAdjustmentLogic/1(ConditionCheck)
  Relational Operator2/1 -> AND2/1
  AND2/1 -> Relational Operator5/1
  Mode_Check/1 -> Relational Operator2/1
  CushionAdjustMode/1 -> Relational Operator2/2
  CushionAdjust/1 -> AND2/2
  Constant2/1 -> Relational Operator5/2

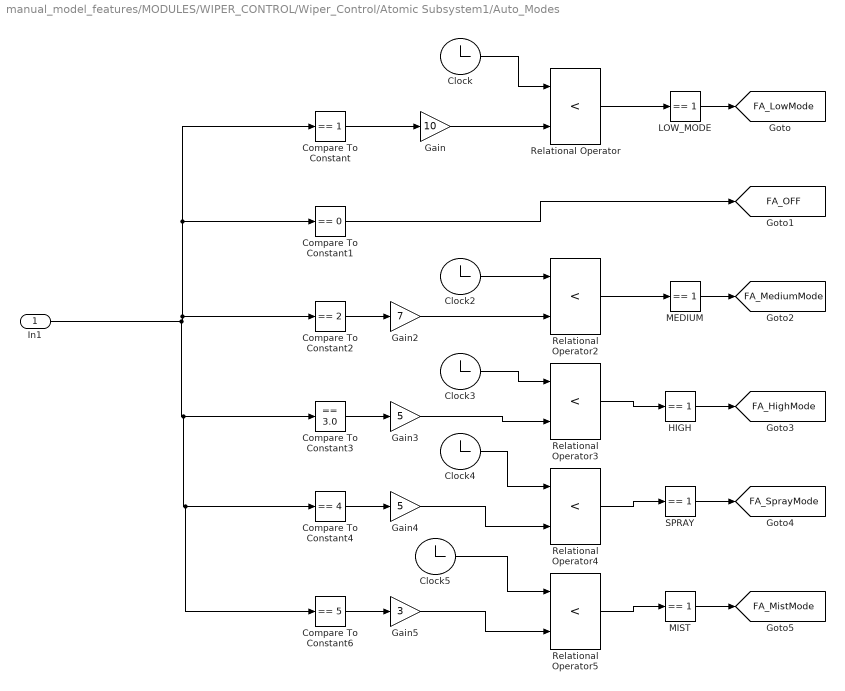
== system manual_model_features/MODULES/WIPER_CONTROL/Wiper_Control/Atomic Subsystem1/Auto_Modes ==
  In1 : Inport
  Clock{,2..5} (5 alike) : Clock
      settings: Decimation=5
  Compare To Constant : simulink/Logic and Bit Operations/Compare To Constant  relop===  const=1  OutDataTypeStr=boolean
  Compare To Constant1 : simulink/Logic and Bit Operations/Compare To Constant  relop===  const=0  OutDataTypeStr=boolean
  Compare To Constant2 : simulink/Logic and Bit Operations/Compare To Constant  relop===  const=2  OutDataTypeStr=boolean
  Compare To Constant3 : simulink/Logic and Bit Operations/Compare To Constant  relop===  const=3.0  OutDataTypeStr=boolean
  Compare To Constant4 : simulink/Logic and Bit Operations/Compare To Constant  relop===  const=4  OutDataTypeStr=boolean
  Compare To Constant6 : simulink/Logic and Bit Operations/Compare To Constant  relop===  const=5  OutDataTypeStr=boolean
  Gain : Gain  Gain=10
  Gain2 : Gain  Gain=7
  Gain3 : Gain  Gain=5
  Gain4 : Gain  Gain=5
  Gain5 : Gain  Gain=3
  HIGH : simulink/Logic and Bit Operations/Compare To Constant  relop===  const=1  OutDataTypeStr=boolean
  LOW_MODE : simulink/Logic and Bit Operations/Compare To Constant  relop===  const=1  OutDataTypeStr=boolean
  MEDIUM : simulink/Logic and Bit Operations/Compare To Constant  relop===  const=1  OutDataTypeStr=boolean
  MIST : simulink/Logic and Bit Operations/Compare To Constant  relop===  const=1  OutDataTypeStr=boolean
  Relational Operator{,2..5} (5 alike) : RelationalOperator  Operator=<  OutDataTypeStr=boolean  RndMeth=Simplest
  SPRAY : simulink/Logic and Bit Operations/Compare To Constant  relop===  const=1  OutDataTypeStr=boolean
  tag scope: FA_HighMode=global, FA_LowMode=global, FA_MediumMode=global, FA_MistMode=global, FA_OFF=global, FA_SprayMode=global
  wires:
  In1/1 -> Compare To Constant6/1, Compare To Constant4/1, Compare To Constant3/1, Compare To Constant2/1, Compare To Constant/1, Compare To Constant1/1
  Clock/1 -> Relational Operator/1
  Relational Operator/1 -> LOW_MODE/1
  Gain/1 -> Relational Operator/2
  Compare To Constant/1 -> Gain/1
  Clock2/1 -> Relational Operator2/1
  Gain2/1 -> Relational Operator2/2
  Compare To Constant2/1 -> Gain2/1
  Clock3/1 -> Relational Operator3/1
  Gain3/1 -> Relational Operator3/2
  Compare To Constant3/1 -> Gain3/1
  Gain4/1 -> Relational Operator4/2
  Clock4/1 -> Relational Operator4/1
  Compare To Constant4/1 -> Gain4/1
  LOW_MODE/1 -> [FA_LowMode]
  MEDIUM/1 -> [FA_MediumMode]
  Relational Operator2/1 -> MEDIUM/1
  HIGH/1 -> [FA_HighMode]
  Relational Operator3/1 -> HIGH/1
  SPRAY/1 -> [FA_SprayMode]
  Relational Operator4/1 -> SPRAY/1
  Compare To Constant1/1 -> [FA_OFF]
  Relational Operator5/1 -> MIST/1
  Gain5/1 -> Relational Operator5/2
  Clock5/1 -> Relational Operator5/1
  MIST/1 -> [FA_MistMode]
  Compare To Constant6/1 -> Gain5/1

== system manual_model_features/MODULES/WIPER_CONTROL/Wiper_Control/Atomic Subsystem1/Manual_mode ==
  In1 : Inport
  Bw30_60 : Logic  IconShape=distinctive  AllPortsSameDT=off  OutDataTypeStr=boolean
  Bw60_100 : Logic  IconShape=distinctive  AllPortsSameDT=off  OutDataTypeStr=boolean
  Compare To Constant1 : simulink/Logic and Bit Operations/Compare To Constant  relop=>  const=30  OutDataTypeStr=boolean
  Compare To Constant2 : simulink/Logic and Bit Operations/Compare To Constant  relop=<=  const=60  OutDataTypeStr=boolean
  Compare To Constant3 : simulink/Logic and Bit Operations/Compare To Constant  relop=>  const=60  OutDataTypeStr=boolean
  Compare To Constant4 : simulink/Logic and Bit Operations/Compare To Constant  relop=<=  const=100  OutDataTypeStr=boolean
  Display : Display
  LessThan30 : simulink/Logic and Bit Operations/Compare To Constant  relop=<=  const=30  OutDataTypeStr=boolean
  Slider : SliderBlock
  String Constant : StringConstant  String="\"Undefined!\""
  Switch : Switch  Criteria=u2 > Threshold  Threshold=5
  tag scope: FM_Bw30_60=global, FM_Bw60_100=global, FM_lessthan30=global
  wires:
  Compare To Constant1/1 -> Bw30_60/1
  Bw30_60/1 -> [FM_Bw30_60]
  [FC_ManualInput] -> Compare To Constant4/1, Compare To Constant3/1, Compare To Constant2/1, Compare To Constant1/1, LessThan30/1, Switch/1
  Compare To Constant4/1 -> Bw60_100/2
  LessThan30/1 -> [FM_lessthan30]
  Switch/1 -> Display/1
  Compare To Constant3/1 -> Bw60_100/1
  Bw60_100/1 -> [FM_Bw60_100]
  Compare To Constant2/1 -> Bw30_60/2
  In1/1 -> Switch/2
  String Constant/1 -> Switch/3
